simulink model "RP_Sumo_Gamepads"  (R2018a)
settings: Solver=ode23t  StartTime=0.0  StopTime=inf  FixedStep=0.05  RelTol=1e-3  EnableMultiTasking=on
InitFcn:
  | RPInit
libraries: RoboticsPlayground x5, vexarmcortexlib x3, vrlib x1
settings Model: EnablePacing=on  ExtModeTrigDuration=25  Creator=scastro  LastModifiedBy=josea
settings SolverCC: AlgebraicLoopSolver=LineSearch
settings DataIOCC: LimitDataPoints=on
settings OptimizationCC: PassReuseOutputArgsAs=Individual arguments  MaxStackSize=64
settings DebuggingCC: ParameterTunabilityLossMsg=error  UnconnectedLineMsg=none  AllowSymbolicDim=off  SFUnexpectedBacktrackingDiag=warning  SFNoUnconditionalDefaultTransitionDiag=warning  SFExecutionAtInitializationDiag=none
settings HardwareCC: ProdBitPerPointer=32  ProdBitPerSizeT=32  ProdBitPerPtrDiffT=32  ProdLargestAtomicInteger=Long  ProdLargestAtomicFloat=Double  ProdWordSize=32  ProdHWDeviceType=ARM Compatible->ARM Cortex
settings SFSimCC: MATLABDynamicMemAlloc=off
settings RTWCC: SystemTargetFile=ert.tlc  HardwareBoard=ARM Cortex-based VEX Microcontroller  TLCOptions="-aInlineSetEventsForThisBaseRateFcn=TLC_FALSE -aSuppressMultiTaskScheduler=TLC_FALSE  -aRateBasedStepFcn=0"  TemplateMakefile=ert_default_tmf  GenerateReport=on  Toolchain=GNU Tools for VEX ARM Cortex  IncludeHyperlinkInReport=on  LaunchReport=on  GenerateTraceInfo=on  GenerateTraceReport=on  GenerateTraceReportSl=on  GenerateTraceReportSf=on  GenerateTraceReportEml=on
settings CodeAppCC: ForceParamTrailComments=on  IgnoreCustomStorageClasses=off  OperatorAnnotations=on  SimulinkDataObjDesc=on  SFDataObjDesc=on  InsertBlockDesc=on
settings ConfigComp: CovMetricSettings=dw  CovHtmlReporting=on  CovSaveCumulativeToWorkspaceVar=on  CovSaveSingleToWorkspaceVar=on  CovExternalEMLEnable=off  CovSFcnEnable=off
settings SimscapeCC: SimscapeNominalValues="[{\"value\":\"10\",\"unit\":\"V\"},{\"value\":\"1\",\"unit\":\"A\"},{\"value\":\"10\",\"unit\":\"N*m\"},{\"value\":\"10\",\"unit\":\"bar\"},{\"value\":\"100\",\"unit\":\"kJ/kg\"},{\"value\":\"1\",\"unit\":\"kW\"},{\"value\":\"300\",\"unit\":\"K\"},{\"value\":\"100\",\"unit\":\"cm^3/s\"},{\"value\":\"1\",\"unit\":\"kN\"},{\"value\":\"1\",\"unit\":\"g/cm^3\"},{\"value\":\"1\",\"unit\":\"l\"},{\"value\":\"1\",\"unit\":\"cm^2\"},{\"value\":\"60\",\"unit\":\"Hz\"}]"  SimscapeLogOpenViewer=on  SimscapeLogLimitData=off  SimscapeLogDataHistory=10000
settings ConfigurationSet: Description=SimMechanics 2G
settings DiagnosticsConfigSet: SimMechanicsRigidlyBoundBlock=none
settings ExplorerConfigSet: InternalSimMechanicsExplorerSettings="<ExplorerConfiguration><canonicalview>default</canonicalview><AnimationSetting><BasePlaybackSpeed>1.0</BasePlaybackSpeed><PlaybackSpeedFactor>1.0</PlaybackSpeedFactor></AnimationSetting><TilePanel><TileInfo><Tiles Columns=\"1\" Count=\"1\" Rows=\"1\"><Column Weight=\"1\"/><Row Weight=\"1\"/><Tile Height=\"1\" Width=\"1\" X=\"0\" Y=\"0\"/></Tiles></TileInfo><SceneInfo><SceneViewer><BGColor><R>0.60000002384185791</R><G>0.60000002384185791</G><B>0.60000002384185791</B></BGColor><Camera><DoPerspective>off</DoPerspective><Position><X>3.46540117628362099</X><Y>-4.48851086982872793</Y><Z>4.67527935374708381</Z></Position><Center><X>-0.00318824384245883219</X><Y>0.0743826421051177328</Y><Z>-0.042399806737498838</Z></Center><Up><X>-0.411121559241908907</X><Y>0.485309543248861219</Y><Z>0.771656471986132075</Z></Up><ViewLimDist>1</ViewLimDist><YLim>2.29173345008683382</YLim><XLim>4.12888596934658469</XLim></Camera></SceneViewer></SceneInfo></TilePanel><MechEditorPanel><Cameras/><GfxPanelCameraMap/><VideoCreator><PlaybackSpeedRatio>1.0</PlaybackSpeedRatio><FrameRate>30</FrameRate><VideoFormat>Motion JPEG AVI</VideoFormat><FrameSize>auto</FrameSize></VideoCreator></MechEditorPanel></ExplorerConfiguration>"

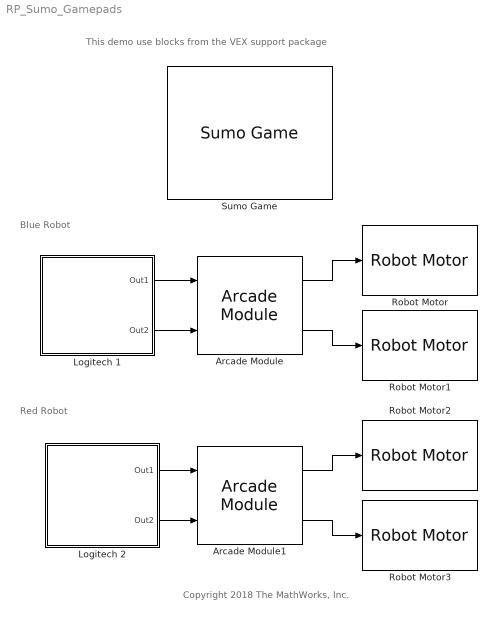
== system RP_Sumo_Gamepads ==
  note: Red Robot
  note: Blue Robot
  note: This demo use blocks from the VEX support package
  note: Copyright 2018 The MathWorks, Inc.
  Arcade Module : vexarmcortexlib/Utilities/Arcade Module
      settings: SourceProductName=Simulink Coder Support Package for ARM Cortex-based VEX Microcontroller  SourceProductBaseCode=EC_VEX_MICRO
  Arcade Module1 : vexarmcortexlib/Utilities/Arcade Module
      settings: SourceProductName=Simulink Coder Support Package for ARM Cortex-based VEX Microcontroller  SourceProductBaseCode=EC_VEX_MICRO
  Logitech 1 : Subsystem
      mask Display:
      | pic = imread('Gamepad_Controller.png');
      | image(pic);
  Logitech 2 : Subsystem
      mask Display:
      | pic = imread('Gamepad_Controller.png');
      | image(pic);
  Robot Motor : RoboticsPlayground/Basic Sensors and Actuators/Robot Motor  OverrideUsingVariant=Rbt1R  robotId=1  motorChoice=2
      settings: SourceProductName=Robotics Playground
  Robot Motor1 : RoboticsPlayground/Basic Sensors and Actuators/Robot Motor  OverrideUsingVariant=Rbt1R  robotId=1  motorChoice=1
      settings: SourceProductName=Robotics Playground
  Robot Motor2 : RoboticsPlayground/Basic Sensors and Actuators/Robot Motor  OverrideUsingVariant=Rbt1R  robotId=2  motorChoice=2
      settings: SourceProductName=Robotics Playground
  Robot Motor3 : RoboticsPlayground/Basic Sensors and Actuators/Robot Motor  OverrideUsingVariant=Rbt1R  robotId=2  motorChoice=1
      settings: SourceProductName=Robotics Playground
  Sumo Game : RoboticsPlayground/Environments/Sumo Game  arenaLength=5  arenaWidth=5  circleRadius=1.8  difficulty=Easy  robot1Id=1  startPose1=[-0.4 0]  wheelBase1=0.5  wheelRadius1=0.1  color1=[0 0 0.5]  robot2Id=2  startPose2=[0.4 0]  wheelBase2=0.5  wheelRadius2=0.1  color2=[0.5 0 0]
      settings: SourceProductName=Robotics Playground
  wires:
  Logitech 1/1(Out1) -> Arcade Module/1
  Logitech 1/2(Out2) -> Arcade Module/2
  Logitech 2/1(Out1) -> Arcade Module1/1
  Logitech 2/2(Out2) -> Arcade Module1/2
  Arcade Module/1 -> Robot Motor/1
  Arcade Module/2 -> Robot Motor1/1
  Arcade Module1/1 -> Robot Motor2/1
  Arcade Module1/2 -> Robot Motor3/1

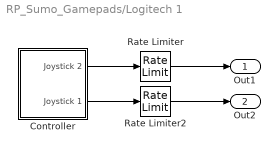
== system RP_Sumo_Gamepads/Logitech 1 ==
  Controller : Subsystem
  Rate Limiter : RateLimiter  RisingSlewLimit=1.2*127  FallingSlewLimit=-1.2*127  SampleTimeMode=inherited
  Rate Limiter2 : RateLimiter  RisingSlewLimit=1.2*127  FallingSlewLimit=-1.2*127  SampleTimeMode=inherited
  Out1 : Outport
  Out2 : Outport  Port=2
  wires:
  Rate Limiter2/1 -> Out2/1
  Rate Limiter/1 -> Out1/1
  Controller/2(Joystick 1) -> Rate Limiter2/1
  Controller/1(Joystick 2) -> Rate Limiter/1

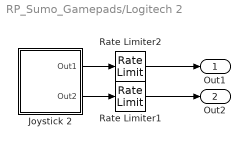
== system RP_Sumo_Gamepads/Logitech 2 ==
  Joystick 2 : Subsystem
  Rate Limiter1 : RateLimiter  RisingSlewLimit=1.2*127  FallingSlewLimit=-1.2*127  SampleTimeMode=inherited
  Rate Limiter2 : RateLimiter  RisingSlewLimit=1.2*127  FallingSlewLimit=-1.2*127  SampleTimeMode=inherited
  Out1 : Outport
  Out2 : Outport  Port=2
  wires:
  Rate Limiter1/1 -> Out2/1
  Rate Limiter2/1 -> Out1/1
  Joystick 2/1(Out1) -> Rate Limiter2/1
  Joystick 2/2(Out2) -> Rate Limiter1/1

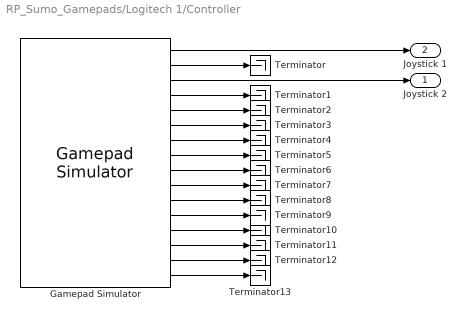
== system RP_Sumo_Gamepads/Logitech 1/Controller ==
  Gamepad Simulator : vexarmcortexlib/Utilities/Gamepad Simulator  WhichPad=Logitech Gamepad  JoyId=1
      settings: SourceProductName=Simulink Coder Support Package for ARM Cortex-based VEX Microcontroller  SourceProductBaseCode=EC_VEX_MICRO
  Terminator{,1..13} (14 alike) : Terminator
  Joystick 2 : Outport
  Joystick 1 : Outport  Port=2
  wires:
  Gamepad Simulator/3 -> Joystick 2/1
  Gamepad Simulator/1 -> Joystick 1/1
  Gamepad Simulator/2 -> Terminator/1
  Gamepad Simulator/4 -> Terminator1/1
  Gamepad Simulator/5 -> Terminator2/1
  Gamepad Simulator/6 -> Terminator3/1
  Gamepad Simulator/7 -> Terminator4/1
  Gamepad Simulator/8 -> Terminator5/1
  Gamepad Simulator/9 -> Terminator6/1
  Gamepad Simulator/10 -> Terminator7/1
  Gamepad Simulator/11 -> Terminator8/1
  Gamepad Simulator/12 -> Terminator9/1
  Gamepad Simulator/13 -> Terminator10/1
  Gamepad Simulator/14 -> Terminator11/1
  Gamepad Simulator/15 -> Terminator12/1
  Gamepad Simulator/16 -> Terminator13/1

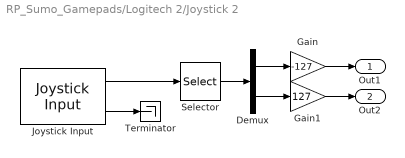
== system RP_Sumo_Gamepads/Logitech 2/Joystick 2 ==
  Demux : Demux  Outputs=2
  Gain : Gain  Gain=-127
  Gain1 : Gain  Gain=127
  Joystick Input : vrlib/Joystick Input  joyid=2  adjustports=on  forcefeed=off
      settings: SourceProductBaseCode=VR
  Selector : Selector  InputPortWidth=4  IndexOptions=Index vector (dialog)  Indices=[2 3]  OutputSizes=1
  Terminator : Terminator
  Out1 : Outport
  Out2 : Outport  Port=2
  wires:
  Gain1/1 -> Out2/1
  Gain/1 -> Out1/1
  Demux/2 -> Gain1/1
  Demux/1 -> Gain/1
  Selector/1 -> Demux/1
  Joystick Input/1 -> Selector/1
  Joystick Input/2 -> Terminator/1
